simulink model "fuzzy_logic_based_model"  (R2021a)
settings: Solver=VariableStepAuto  StartTime=0.0  StopTime=100  RelTol=1e-3
libraries: fuzblock x4
settings Model: SimulationMode=accelerator  Creator=uddin  LastModifiedBy=uddin

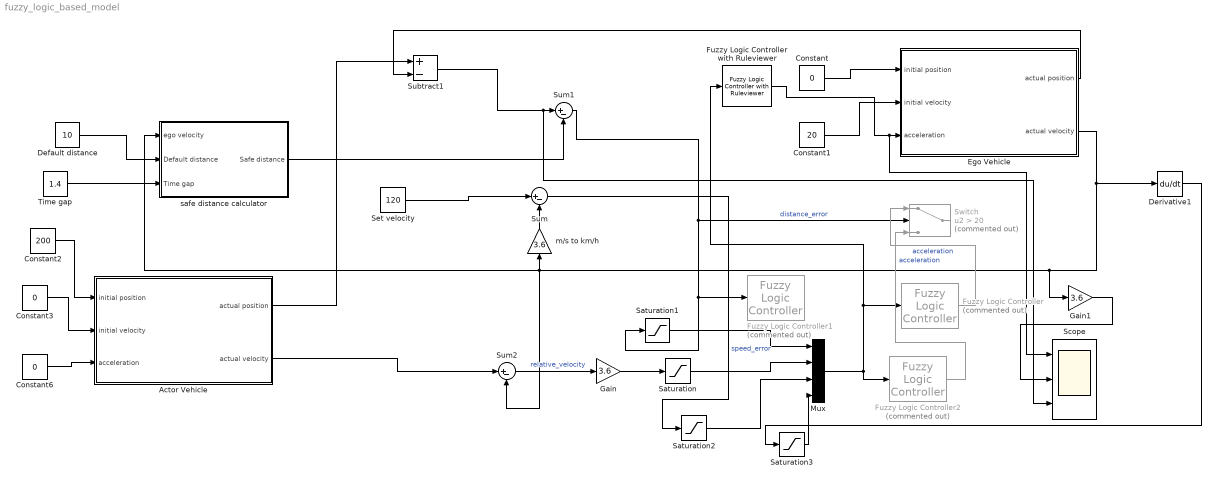
== system fuzzy_logic_based_model ==
  Actor Vehicle : Subsystem
  Constant : Constant  Value=0  SampleTime=.1
  Constant1 : Constant  Value=20  SampleTime=.1
  Constant2 : Constant  Value=200  SampleTime=.1
  Constant3 : Constant  Value=0  SampleTime=.1
  Constant6 : Constant  Value=0  SampleTime=.1
  Default distance : Constant  Value=10  SampleTime=.1
  Derivative1 : Derivative
  Ego Vehicle : Subsystem
  Fuzzy Logic Controller : fuzblock/Fuzzy Logic  Controller  Commented=on  FIS=fisi  OutputSampleNumber=101  DataType=double  FuzzifiedInputs=off  RuleFiringStrengths=off  RuleOutputs=off  AggregatedOutputs=off  SimulateUsing=Interpreted execution  OutOfRangeInputValueMessage=warning  NoRuleFiredMessage=warning  EmptyOutputFuzzySetMessage=warning
  Fuzzy Logic Controller with Ruleviewer : fuzblock/Fuzzy Logic  Controller  with Ruleviewer  fismatrix=fis  Ts=2
  Fuzzy Logic Controller1 : fuzblock/Fuzzy Logic  Controller  Commented=on  FIS=taken  OutputSampleNumber=101  DataType=double  FuzzifiedInputs=off  RuleFiringStrengths=off  RuleOutputs=off  AggregatedOutputs=off  SimulateUsing=Interpreted execution  OutOfRangeInputValueMessage=warning  NoRuleFiredMessage=warning  EmptyOutputFuzzySetMessage=warning
  Fuzzy Logic Controller2 : fuzblock/Fuzzy Logic  Controller  Commented=on  FIS=fisr  OutputSampleNumber=101  DataType=double  FuzzifiedInputs=off  RuleFiringStrengths=off  RuleOutputs=off  AggregatedOutputs=off  SimulateUsing=Interpreted execution  OutOfRangeInputValueMessage=warning  NoRuleFiredMessage=warning  EmptyOutputFuzzySetMessage=warning
  Gain : Gain  Gain=3.6
  Gain1 : Gain  Gain=3.6
  Mux : Mux
  Saturation{,1..3} (4 alike) : Saturate  UpperLimit=1  LowerLimit=-1  LinearizeAsGain=off
  Scope : Scope  NumInputPorts=3
  Set velocity : Constant  Value=120  SampleTime=.1
  Subtract1 : Sum  Inputs=+-
  Sum : Sum  Inputs=|+-
  Sum1 : Sum  Inputs=|+-
  Sum2 : Sum  Inputs=|+-
  Switch : Switch  Commented=on  Criteria=u2 > Threshold  Threshold=20
  Time gap : Constant  Value=1.4  SampleTime=.1
  m/s to km/h : Gain  Gain=3.6
  safe distance calculator : Subsystem
  wires:
  Time gap/1 -> safe distance calculator/3(Time gap)
  Default distance/1 -> safe distance calculator/2(Default distance)
  Constant2/1 -> Actor Vehicle/1(initial position)
  Constant3/1 -> Actor Vehicle/2(initial velocity)
  Constant6/1 -> Actor Vehicle/3(acceleration)
  Constant/1 -> Ego Vehicle/1(initial position)
  Constant1/1 -> Ego Vehicle/2(initial velocity)
  safe distance calculator/1(Safe distance) -> Sum1/2
  Actor Vehicle/1(actual position) -> Subtract1/1
  Ego Vehicle/1(actual position) -> Subtract1/2
  Subtract1/1 -> Scope/3, Sum1/1
  Actor Vehicle/2(actual velocity) -> Sum2/1
  Sum1/1 -> Switch/2, Fuzzy Logic Controller1/1, Saturation1/1  "distance_error"
  Sum/1 -> Saturation2/1  "speed_error"
  Set velocity/1 -> Sum/1
  m/s to km/h/1 -> Sum/2
  Sum2/1 -> Gain/1  "relative_velocity"
  Gain1/1 -> Scope/2
  Mux/1 -> Fuzzy Logic Controller2/1, Fuzzy Logic Controller with Ruleviewer/1, Fuzzy Logic Controller/1
  Ego Vehicle/2(actual velocity) -> Sum2/2, safe distance calculator/1(ego velocity), m/s to km/h/1, Gain1/1, Derivative1/1
  Fuzzy Logic Controller/1 -> Switch/1  "acceleration"
  Fuzzy Logic Controller2/1 -> Switch/3  "acceleration"
  Fuzzy Logic Controller with Ruleviewer/1 -> Scope/1, Ego Vehicle/3(acceleration)
  Gain/1 -> Saturation/1
  Saturation/1 -> Mux/2
  Saturation1/1 -> Mux/1
  Saturation2/1 -> Mux/3
  Derivative1/1 -> Saturation3/1
  Saturation3/1 -> Mux/4

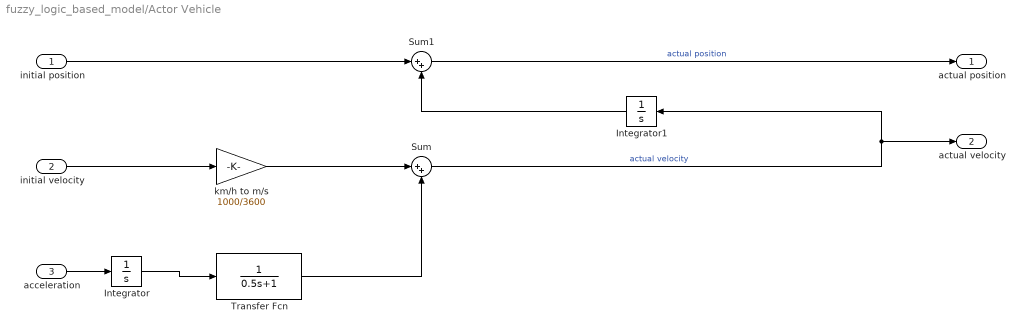
== system fuzzy_logic_based_model/Actor Vehicle ==
  initial position : Inport
  initial velocity : Inport  Port=2
  acceleration : Inport  Port=3
  Integrator : Integrator
  Integrator1 : Integrator
  Sum : Sum  Inputs=|++
  Sum1 : Sum  Inputs=|++
  Transfer Fcn : TransferFcn  Denominator=[0.5 1]
  km/h to m/s : Gain  Gain=1000/3600
  actual position : Outport
  actual velocity : Outport  Port=2
  wires:
  km/h to m/s/1 -> Sum/1
  initial velocity/1 -> km/h to m/s/1
  Transfer Fcn/1 -> Sum/2
  Integrator/1 -> Transfer Fcn/1
  Integrator1/1 -> Sum1/2
  initial position/1 -> Sum1/1
  acceleration/1 -> Integrator/1
  Sum/1 -> Integrator1/1, actual velocity/1  "actual velocity"
  Sum1/1 -> actual position/1  "actual position"

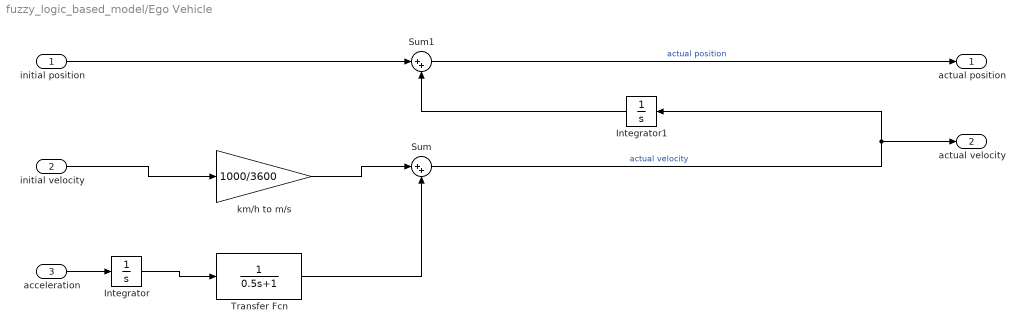
== system fuzzy_logic_based_model/Ego Vehicle ==
  initial position : Inport
  initial velocity : Inport  Port=2
  acceleration : Inport  Port=3
  Integrator : Integrator
  Integrator1 : Integrator
  Sum : Sum  Inputs=|++
  Sum1 : Sum  Inputs=|++
  Transfer Fcn : TransferFcn  Denominator=[0.5 1]
  km/h to m/s : Gain  Gain=1000/3600
  actual position : Outport
  actual velocity : Outport  Port=2
  wires:
  Sum1/1 -> actual position/1  "actual position"
  Sum/1 -> actual velocity/1, Integrator1/1  "actual velocity"
  acceleration/1 -> Integrator/1
  initial position/1 -> Sum1/1
  Integrator1/1 -> Sum1/2
  Integrator/1 -> Transfer Fcn/1
  Transfer Fcn/1 -> Sum/2
  initial velocity/1 -> km/h to m/s/1
  km/h to m/s/1 -> Sum/1

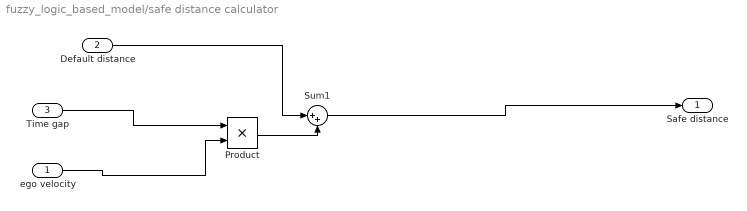
== system fuzzy_logic_based_model/safe distance calculator ==
  ego velocity : Inport
  Default distance : Inport  Port=2
  Time gap : Inport  Port=3
  Product : Product
  Sum1 : Sum  Inputs=|++
  Safe distance : Outport
  wires:
  Product/1 -> Sum1/2
  Sum1/1 -> Safe distance/1
  Time gap/1 -> Product/1
  Default distance/1 -> Sum1/1
  ego velocity/1 -> Product/2
